simulink model "BuckFeedbackExampleCh9GvgOpenLoop"  (Simulink 7.5)
settings: Solver=ode45  StartTime=0.0  StopTime=10.0  RelTol=1e-3
settings Model: Creator=rwe  LastModifiedBy=rwe

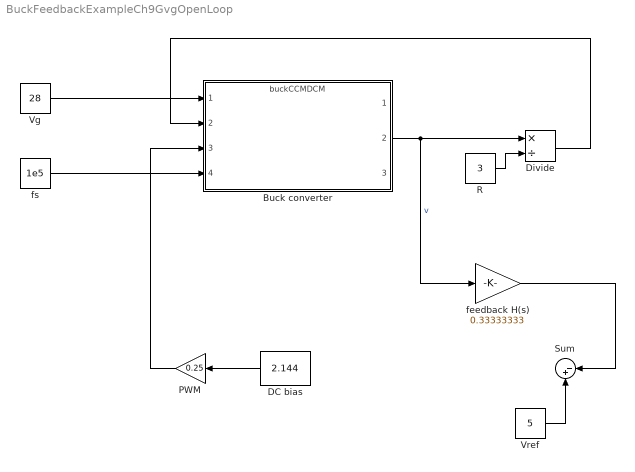
== system BuckFeedbackExampleCh9GvgOpenLoop ==
  Buck converter : ModelReference  ModelNameDialog=buckCCMDCM  SimulationMode=Accelerator  ModelReferenceVersion=1.27  CopyOfModelName=buckCCMDCM
  DC bias : Constant  Value=2.144  OutDataType=fixdt(1, 16)  OutScaling=2^0
  Divide : Product  Inputs=*/  OutDataType=fixdt(1, 16)  OutScaling=2^-10
  PWM : Gain  Gain=0.25  ParameterDataType=fixdt(1, 16)  ParameterScaling=2^0  OutDataType=fixdt(1, 16)  OutScaling=2^0
  R : Constant  Value=3  OutDataType=fixdt(1, 16)  OutScaling=2^0
  Sum : Sum  Inputs=|-+  OutDataType=fixdt(1, 16)  OutScaling=2^0
  Vg : Constant  Value=28  OutDataType=fixdt(1, 16)  OutScaling=2^0
  Vref : Constant  Value=5  OutDataType=fixdt(1, 16)  OutScaling=2^0
  feedback H(s) : Gain  Gain=0.33333333  ParameterDataType=fixdt(1, 16)  ParameterScaling=2^0  OutDataType=fixdt(1, 16)  OutScaling=2^0
  fs : Constant  Value=1e5  OutDataType=fixdt(1, 16)  OutScaling=2^0
  wires:
  Vg/1 -> Buck converter/1
  Buck converter/2 -> Divide/1, feedback H(s)/1  "v"
  Divide/1 -> Buck converter/2
  R/1 -> Divide/2
  fs/1 -> Buck converter/4
  feedback H(s)/1 -> Sum/1
  Vref/1 -> Sum/2
  PWM/1 -> Buck converter/3
  DC bias/1 -> PWM/1
